simulink model "IRIS_fuzzy"  (Simulink 8.5)
settings: Solver=ode45  StartTime=0.0  StopTime=20  MinStep=0.0001  RelTol=1e-3
undefined symbols (not defined in the file or in its folder): quad
libraries: fuzblock x5, simulink x3
settings Model: Creator=evgenov  LastModifiedBy=Alexey
settings DebuggingCC: MaxConsecutiveZCsMsg=warning  SolverPrmCheckMsg=warning  FcnCallInpInsideContextMsg=UseLocalSettings

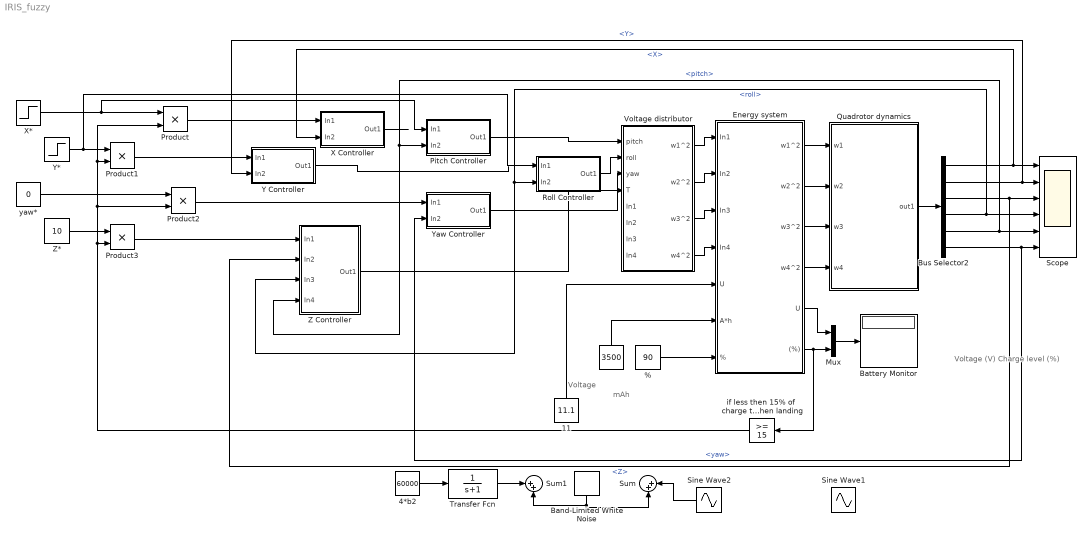
== system IRIS_fuzzy ==
  note: Voltage
  note: Voltage (V)
      |
      | Charge level (%)
  note: mAh
  "  " : Constant  Value=3500
  " 11" : Constant  Value=11.1
  % : Constant  Value=90
  4*b2 : Constant  Value=60000
  Band-Limited White Noise : simulink/Sources/Band-Limited White Noise  Cov=[2000]  Ts=0.1  seed=[23341]
  Battery Monitor : Display
  Bus Selector2 : BusSelector  OutputSignals=X,Y,Z,roll,pitch,yaw
  Energy system : Subsystem
  Mux : Mux  Inputs=2
  Pitch Controller : Subsystem
  Product{,1..3} (4 alike) : Product
  Quadrotor dynamics : Subsystem
  Roll Controller : Subsystem
  Scope : Scope  NumInputPorts=6
      settings: TimeRange=20  YMin=-0.0005~-0.0175~0~-0.025~-0.125~0  YMax=0.0035~0.0025~10~0.125~0.025~1  SaveName=ScopeData2
  Sine Wave1 : Sin  Amplitude=100000  Frequency=0.5  SampleTime=0
  Sine Wave2 : Sin  Amplitude=500000  SampleTime=0
  Sum : Sum  Inputs=|++
  Sum1 : Sum  Inputs=|++
  Transfer Fcn : TransferFcn  Denominator=[1 1]
  Voltage distributor : Subsystem
  X Controller : Subsystem
  X* : Step  Time=5  After=0  SampleTime=0  ZeroCross=off
  Y Controller : Subsystem
  Y* : Step  Time=5  After=0  SampleTime=0  ZeroCross=off
  Yaw Controller : Subsystem
  Z Controller : Subsystem
  Z* : Constant  Value=10
  if less then 15% of  charge then landing : simulink/Logic and Bit Operations/Compare To Constant  relop=>=  const=15  OutDataTypeStr=uint8
  yaw* : Constant  Value=0
  wires:
  Bus Selector2/1 -> X Controller/2(In2), Scope/1  "<X>"
  Bus Selector2/2 -> Y Controller/2(In2), Scope/2  "<Y>"
  Bus Selector2/3 -> Z Controller/2(In2), Scope/3  "<Z>"
  Bus Selector2/4 -> Roll Controller/2(In2), Z Controller/3(In3), Scope/4  "<roll>"
  Bus Selector2/6 -> Yaw Controller/2(In2), Scope/6  "<yaw>"
  Bus Selector2/5 -> Z Controller/4(In4), Pitch Controller/2(In2), Scope/5  "<pitch>"
  Yaw Controller/1(Out1) -> Voltage distributor/3(yaw)
  Roll Controller/1(Out1) -> Voltage distributor/2(roll)
  Pitch Controller/1(Out1) -> Voltage distributor/1(pitch)
  X Controller/1(Out1) -> ?
  "  "/1 -> Energy system/6(A*h)
  " 11"/1 -> Energy system/5(U)
  %/1 -> Energy system/7(%)
  Voltage distributor/1("w1^2 ") -> Energy system/1(In1)
  Voltage distributor/2("w2^2 ") -> Energy system/2(In2)
  Voltage distributor/3("w3^2 ") -> Energy system/3(In3)
  Voltage distributor/4("w4^2 ") -> Energy system/4(In4)
  Energy system/1(w1^2) -> Quadrotor dynamics/1(w1)
  Energy system/2(w2^2) -> Quadrotor dynamics/2(w2)
  Energy system/3(w3^2) -> Quadrotor dynamics/3(w3)
  Energy system/4(w4^2) -> Quadrotor dynamics/4(w4)
  Quadrotor dynamics/1(out1) -> Bus Selector2/1
  Mux/1 -> Battery Monitor/1
  Energy system/5("U ") -> Mux/1
  Energy system/6(" (%)") -> if less then 15% of  charge then landing/1, Mux/2
  X*/1 -> Pitch Controller/1(In1), Product/1
  Product/1 -> X Controller/1(In1)
  Y*/1 -> Roll Controller/1(In1), Product1/1
  Product1/1 -> Y Controller/1(In1)
  Product2/1 -> Yaw Controller/1(In1)
  Product3/1 -> Z Controller/1(In1)
  if less then 15% of  charge then landing/1 -> Product3/2, Product2/2, Product1/2, Product/2
  Z Controller/1(Out1) -> Voltage distributor/4(T)
  Y Controller/1(Out1) -> ?
  4*b2/1 -> Transfer Fcn/1
  Transfer Fcn/1 -> Sum1/1
  Sine Wave2/1 -> Sum/1
  Band-Limited White Noise/1 -> Sum1/2, Sum/2
  yaw*/1 -> Product2/1
  Z*/1 -> Product3/1

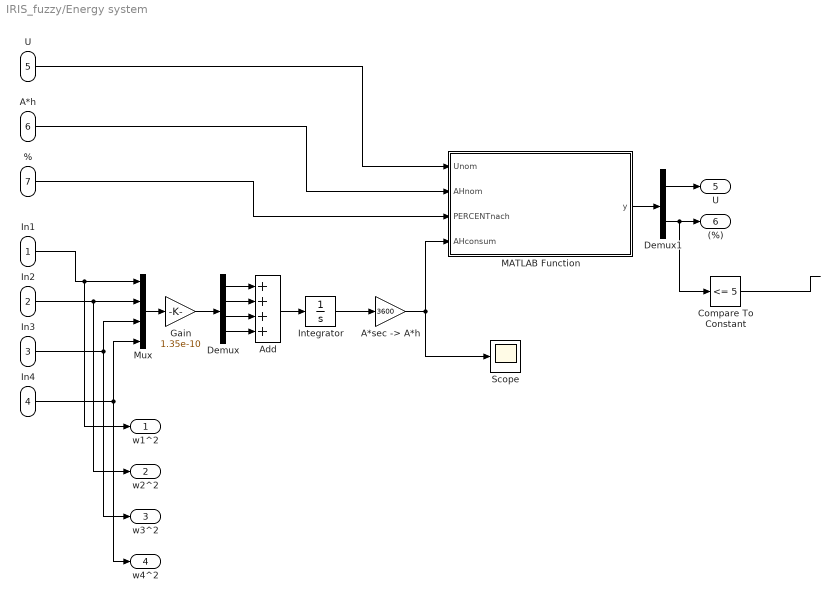
== system IRIS_fuzzy/Energy system ==
  In1 : Inport
  In2 : Inport  Port=2
  In3 : Inport  Port=3
  In4 : Inport  Port=4
  U : Inport  Port=5
  A*h : Inport  Port=6
  % : Inport  Port=7
  "A*sec -> A*h" : Gain  Gain=3600
  Add : Sum  Inputs=++++
  Compare To Constant : simulink/Logic and Bit Operations/Compare To Constant  relop=<=  const=5  OutDataTypeStr=uint8
  Demux : Demux
  Demux1 : Demux  Outputs=2
  Gain : Gain  Gain=1.35e-10
  Integrator : Integrator
  MATLAB Function : MATLAB Function  TreatAsAtomicUnit=on
  Mux : Mux
  Scope : Scope
  w1^2 : Outport
  w2^2 : Outport  Port=2
  w3^2 : Outport  Port=3
  w4^2 : Outport  Port=4
  "U " : Outport  Port=5
  " (%)" : Outport  Port=6
  wires:
  Add/1 -> Integrator/1
  Gain/1 -> Demux/1
  Demux/2 -> Add/2
  Integrator/1 -> "A*sec -> A*h"/1
  Mux/1 -> Gain/1
  In4/1 -> Mux/4, w4^2/1
  In2/1 -> w2^2/1, Mux/2
  Demux/1 -> Add/1
  Demux/4 -> Add/4
  Demux/3 -> Add/3
  In1/1 -> w1^2/1, Mux/1
  In3/1 -> Mux/3, w3^2/1
  U/1 -> MATLAB Function/1(Unom)
  A*h/1 -> MATLAB Function/2(AHnom)
  %/1 -> MATLAB Function/3(PERCENTnach)
  "A*sec -> A*h"/1 -> MATLAB Function/4(AHconsum), Scope/1
  MATLAB Function/1(y) -> Demux1/1
  Demux1/1 -> "U "/1
  Demux1/2 -> Compare To Constant/1, " (%)"/1
  Compare To Constant/1 -> ?

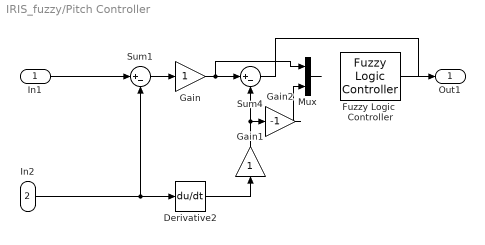
== system IRIS_fuzzy/Pitch Controller ==
  In1 : Inport
  In2 : Inport  Port=2
  Derivative2 : Derivative
  Fuzzy Logic  Controller : fuzblock/Fuzzy Logic  Controller  fis='FuzzyPD roll pitch.fis'
  Gain : Gain
  Gain1 : Gain
  Gain2 : Gain  Gain=-1
  Mux : Mux  Inputs=2
  Sum1 : Sum  Inputs=|+-
  Sum4 : Sum  Inputs=|+-
  Out1 : Outport
  wires:
  In1/1 -> Sum1/1
  In2/1 -> Derivative2/1, Sum1/2
  Sum1/1 -> Gain/1
  Gain/1 -> Sum4/1, Mux/1
  Derivative2/1 -> Gain1/1
  Gain1/1 -> Sum4/2, Gain2/1
  Mux/1 -> ?
  Fuzzy Logic  Controller/1 -> ?
  Gain2/1 -> Mux/2
  Sum4/1 -> Out1/1

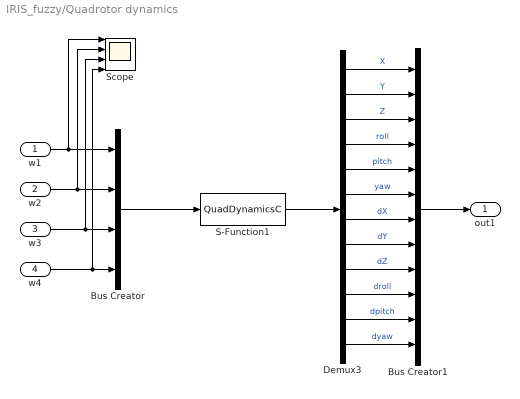
== system IRIS_fuzzy/Quadrotor dynamics ==
  w1 : Inport
  w2 : Inport  Port=2
  w3 : Inport  Port=3
  w4 : Inport  Port=4
  Bus Creator : BusCreator
  Bus Creator1 : BusCreator  Inputs=12
  Demux3 : Demux  Outputs=12
  S-Function1 : S-Function  FunctionName=QuadDynamicsC  Parameters=quad
  Scope : Scope  NumInputPorts=4
      settings: YMin=-5~-5~-5~-5  YMax=5~5~5~5
  out1 : Outport
  wires:
  w1/1 -> Scope/1, Bus Creator/1
  w2/1 -> Scope/2, Bus Creator/2
  w3/1 -> Scope/3, Bus Creator/3
  w4/1 -> Scope/4, Bus Creator/4
  Bus Creator1/1 -> out1/1
  Bus Creator/1 -> S-Function1/1
  Demux3/1 -> Bus Creator1/1  "X"
  Demux3/2 -> Bus Creator1/2  "Y"
  Demux3/3 -> Bus Creator1/3  "Z"
  Demux3/4 -> Bus Creator1/4  "roll"
  Demux3/5 -> Bus Creator1/5  "pitch"
  Demux3/6 -> Bus Creator1/6  "yaw"
  Demux3/7 -> Bus Creator1/7  "dX"
  Demux3/8 -> Bus Creator1/8  "dY"
  Demux3/9 -> Bus Creator1/9  "dZ"
  Demux3/10 -> Bus Creator1/10  "droll"
  Demux3/11 -> Bus Creator1/11  "dpitch"
  Demux3/12 -> Bus Creator1/12  "dyaw"
  S-Function1/1 -> Demux3/1

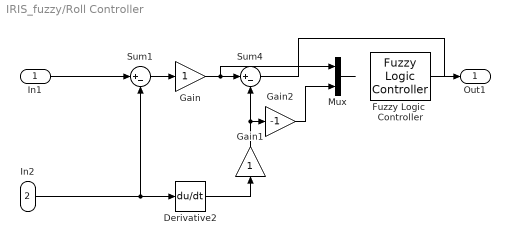
== system IRIS_fuzzy/Roll Controller ==
  In1 : Inport
  In2 : Inport  Port=2
  Derivative2 : Derivative
  Fuzzy Logic  Controller : fuzblock/Fuzzy Logic  Controller  fis='FuzzyPD roll pitch.fis'
  Gain : Gain
  Gain1 : Gain
  Gain2 : Gain  Gain=-1
  Mux : Mux  Inputs=2
  Sum1 : Sum  Inputs=|+-
  Sum4 : Sum  Inputs=|+-
  Out1 : Outport
  wires:
  In1/1 -> Sum1/1
  In2/1 -> Derivative2/1, Sum1/2
  Sum1/1 -> Gain/1
  Gain/1 -> Sum4/1, Mux/1
  Derivative2/1 -> Gain1/1
  Gain1/1 -> Sum4/2, Gain2/1
  Mux/1 -> ?
  Gain2/1 -> Mux/2
  Sum4/1 -> Out1/1
  Fuzzy Logic  Controller/1 -> ?

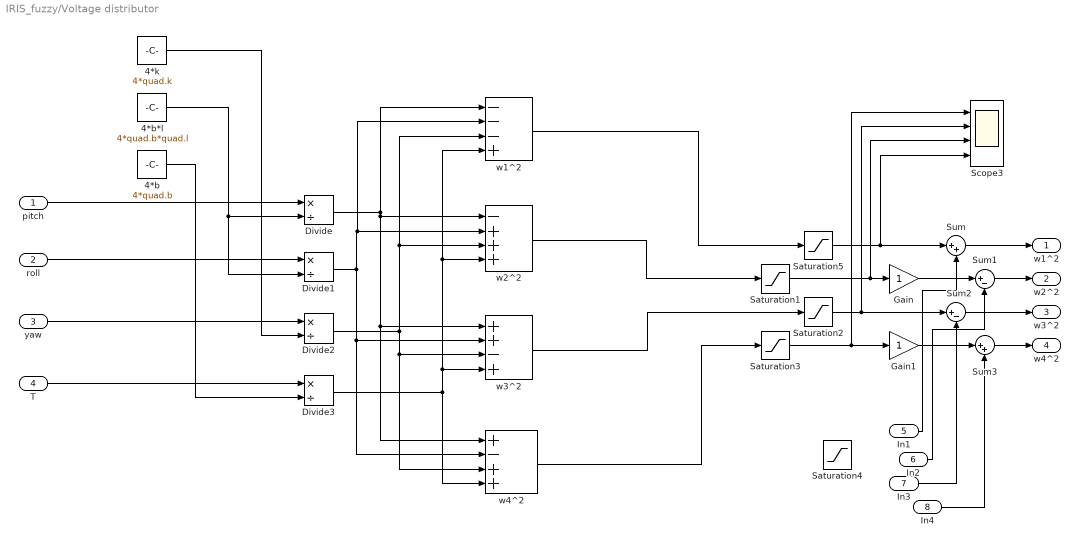
== system IRIS_fuzzy/Voltage distributor ==
  pitch : Inport
  roll : Inport  Port=2
  yaw : Inport  Port=3
  T : Inport  Port=4
  In1 : Inport  Port=5
  In2 : Inport  Port=6
  In3 : Inport  Port=7
  In4 : Inport  Port=8
  4*b : Constant  Value=4*quad.b
  4*b*l : Constant  Value=4*quad.b*quad.l
  4*k : Constant  Value=4*quad.k
  Divide{,1..3} (4 alike) : Product  Inputs=*/
  Gain : Gain
  Gain1 : Gain
  Saturation{1..3,5} (4 alike) : Saturate  UpperLimit=2000^2  LowerLimit=500^2  ZeroCross=off
  Saturation4 : Saturate  UpperLimit=5490^2  LowerLimit=500^2  ZeroCross=off
  Scope3 : Scope  NumInputPorts=4
      settings: YMin=-5~-5~-5~-5  YMax=5~5~5~5  SaveName=ScopeData7
  Sum : Sum  Inputs=|++
  Sum1 : Sum  Inputs=|+-
  Sum2 : Sum  Inputs=|+-
  Sum3 : Sum  Inputs=|++
  w1^2 : Sum  Inputs=---+
  w2^2 : Sum  Inputs=-+++
  w3^2 : Sum  Inputs=++-+
  w4^2 : Sum  Inputs=+-++
  "w1^2 " : Outport
  "w2^2 " : Outport  Port=2
  "w3^2 " : Outport  Port=3
  "w4^2 " : Outport  Port=4
  wires:
  4*k/1 -> Divide2/2
  Divide1/1 -> w3^2/2, w4^2/2, w1^2/2, w2^2/2
  Divide2/1 -> w4^2/3, w3^2/3, w2^2/3, w1^2/3
  Divide/1 -> w2^2/1, w4^2/1, w3^2/1, w1^2/1
  4*b/1 -> Divide3/2
  yaw/1 -> Divide2/1
  4*b*l/1 -> Divide/2, Divide1/2
  roll/1 -> Divide1/1
  pitch/1 -> Divide/1
  Divide3/1 -> w4^2/4, w3^2/4, w2^2/4, w1^2/4
  Saturation5/1 -> Sum/1, Scope3/4
  Saturation1/1 -> Gain/1, Scope3/3
  Saturation2/1 -> Sum2/1, Scope3/2
  Saturation3/1 -> Gain1/1, Scope3/1
  w1^2/1 -> Saturation5/1
  w2^2/1 -> Saturation1/1
  w3^2/1 -> Saturation2/1
  w4^2/1 -> Saturation3/1
  T/1 -> Divide3/1
  Sum/1 -> "w1^2 "/1
  Sum2/1 -> "w3^2 "/1
  Sum1/1 -> "w2^2 "/1
  Gain/1 -> Sum1/1
  In1/1 -> Sum/2
  In2/1 -> Sum1/2
  In3/1 -> Sum2/2
  In4/1 -> Sum3/2
  Sum3/1 -> "w4^2 "/1
  Gain1/1 -> Sum3/1

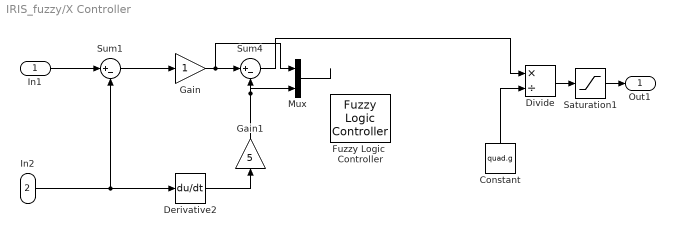
== system IRIS_fuzzy/X Controller ==
  In1 : Inport
  In2 : Inport  Port=2
  Constant : Constant  Value=quad.g
  Derivative2 : Derivative
  Divide : Product  Inputs=*/
  Fuzzy Logic  Controller : fuzblock/Fuzzy Logic  Controller  fis='FuzzyPD z.fis'
  Gain : Gain
  Gain1 : Gain  Gain=5
  Mux : Mux  Inputs=2
  Saturation1 : Saturate  UpperLimit=0.1  LowerLimit=-0.1  ZeroCross=off
  Sum1 : Sum  Inputs=|+-
  Sum4 : Sum  Inputs=|+-
  Out1 : Outport
  wires:
  In2/1 -> Sum1/2, Derivative2/1
  Gain/1 -> Sum4/1, Mux/1
  Derivative2/1 -> Gain1/1
  Gain1/1 -> Sum4/2, Mux/2
  Constant/1 -> Divide/2
  Divide/1 -> Saturation1/1
  Saturation1/1 -> Out1/1
  In1/1 -> Sum1/1
  Sum1/1 -> Gain/1
  ? -> ?
  Mux/1 -> ?
  Sum4/1 -> Divide/1

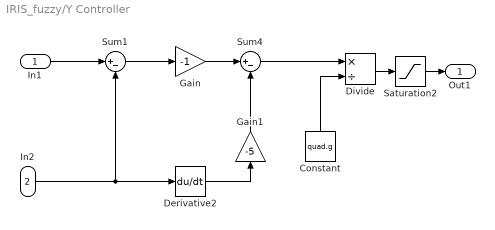
== system IRIS_fuzzy/Y Controller ==
  In1 : Inport
  In2 : Inport  Port=2
  Constant : Constant  Value=quad.g
  Derivative2 : Derivative
  Divide : Product  Inputs=*/
  Gain : Gain  Gain=-1
  Gain1 : Gain  Gain=-5
  Saturation2 : Saturate  UpperLimit=0.1  LowerLimit=-0.1  ZeroCross=off
  Sum1 : Sum  Inputs=|+-
  Sum4 : Sum  Inputs=|+-
  Out1 : Outport
  wires:
  In2/1 -> Sum1/2, Derivative2/1
  Gain/1 -> Sum4/1
  Derivative2/1 -> Gain1/1
  Gain1/1 -> Sum4/2
  Sum4/1 -> Divide/1
  Constant/1 -> Divide/2
  Divide/1 -> Saturation2/1
  Saturation2/1 -> Out1/1
  In1/1 -> Sum1/1
  Sum1/1 -> Gain/1

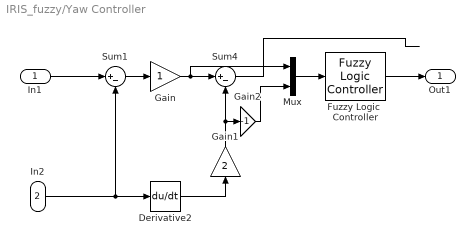
== system IRIS_fuzzy/Yaw Controller ==
  In1 : Inport
  In2 : Inport  Port=2
  Derivative2 : Derivative
  Fuzzy Logic  Controller : fuzblock/Fuzzy Logic  Controller  fis='FuzzyPD yaw.fis'
  Gain : Gain
  Gain1 : Gain  Gain=2
  Gain2 : Gain  Gain=-1
  Mux : Mux  Inputs=2
  Sum1 : Sum  Inputs=|+-
  Sum4 : Sum  Inputs=|+-
  Out1 : Outport
  wires:
  In1/1 -> Sum1/1
  In2/1 -> Derivative2/1, Sum1/2
  Sum1/1 -> Gain/1
  Gain/1 -> Sum4/1, Mux/1
  Derivative2/1 -> Gain1/1
  Gain1/1 -> Sum4/2, Gain2/1
  Mux/1 -> Fuzzy Logic  Controller/1
  Fuzzy Logic  Controller/1 -> Out1/1
  Gain2/1 -> Mux/2
  Sum4/1 -> ?

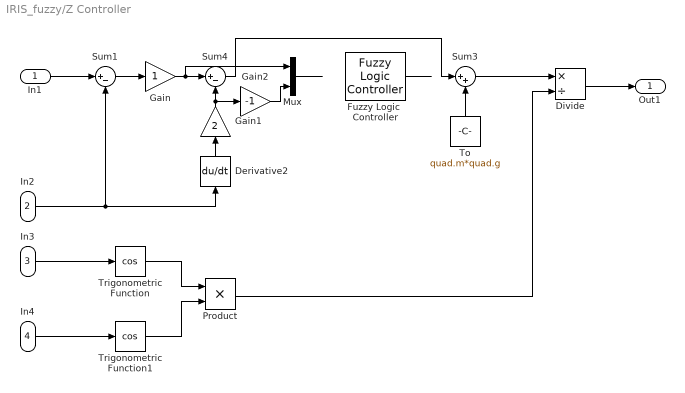
== system IRIS_fuzzy/Z Controller ==
  In1 : Inport
  In2 : Inport  Port=2
  In3 : Inport  Port=3
  In4 : Inport  Port=4
  Derivative2 : Derivative
  Divide : Product  Inputs=*/
  Fuzzy Logic  Controller : fuzblock/Fuzzy Logic  Controller  fis='FuzzyPD z.fis'
  Gain : Gain
  Gain1 : Gain  Gain=2
  Gain2 : Gain  Gain=-1
  Mux : Mux  Inputs=2
  Product : Product
  Sum1 : Sum  Inputs=|+-
  Sum3 : Sum  Inputs=|++
  Sum4 : Sum  Inputs=|+-
  To : Constant  Value=quad.m*quad.g
  Trigonometric Function : Trigonometry  Operator=cos
  Trigonometric Function1 : Trigonometry  Operator=cos
  Out1 : Outport
  wires:
  In4/1 -> Trigonometric Function1/1
  In3/1 -> Trigonometric Function/1
  Trigonometric Function/1 -> Product/1
  Trigonometric Function1/1 -> Product/2
  Product/1 -> Divide/2
  To/1 -> Sum3/2
  Sum3/1 -> Divide/1
  Divide/1 -> Out1/1
  In1/1 -> Sum1/1
  Gain/1 -> Sum4/1, Mux/1
  Derivative2/1 -> Gain1/1
  Gain1/1 -> Sum4/2, Gain2/1
  In2/1 -> Sum1/2, Derivative2/1
  Sum1/1 -> Gain/1
  Fuzzy Logic  Controller/1 -> ?
  Mux/1 -> ?
  Gain2/1 -> Mux/2
  Sum4/1 -> Sum3/1

== matlab function Energy system/MATLAB Function ==
  data: Unom input double; AHnom input double; PERCENTnach input double; AHconsum input double; y output double
function y = fcn(Unom,AHnom,PERCENTnach,AHconsum)
%#codegen
k=0.117*Unom/AHnom;

%  
AH=PERCENTnach*AHnom/100-AHconsum;
% 
U=0.964*Unom+k*AH;
% 
Charge=AH*100/AHnom;

y=[U;Charge]
